simulink model "mpptPandO"  (R2024b)
settings: Solver=VariableStepAuto  StartTime=0.0  StopTime=1  RelTol=1e-3
undefined symbols (not defined in the file): sigbuilder_block
libraries: spsSeriesRLCBranchLib x4, spsCurrentMeasurementLib x1, spsDiodeLib x1, spsMosfetLib x1, spsPWMGeneratorDCDCLib x1, spsPVArrayLib x1, spsVoltageMeasurementLib x1, spspowerguiLib x1
settings Model: Creator=RASITH  LastModifiedBy=RASITH

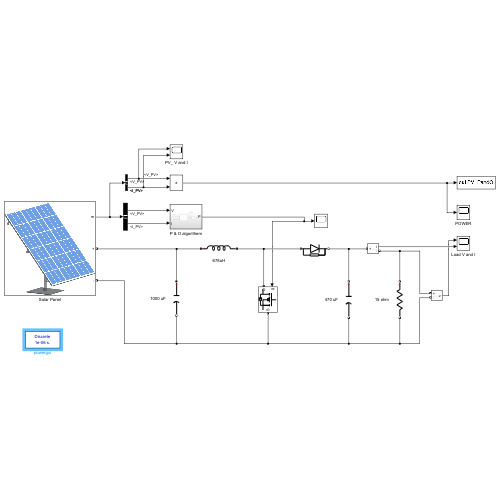
[thumbnail: Simulink's stored preview of the top-level diagram]
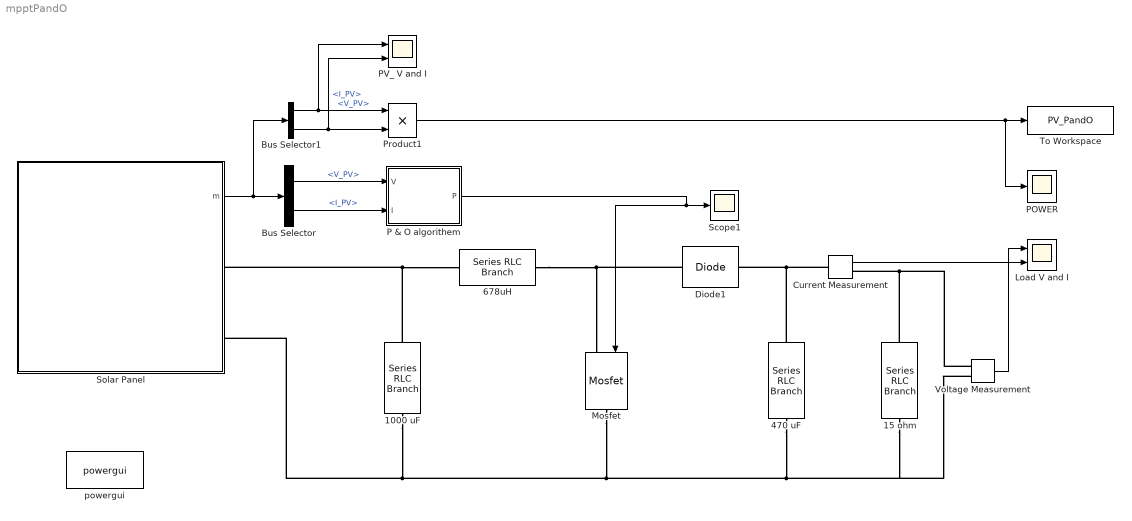
== system mpptPandO ==
  1000 uF : spsSeriesRLCBranchLib/Series RLC Branch  LConnTagsString=__new0  RConnTagsString=__new0  BranchType=C  Resistance=1  Inductance=1e-3  SetiL0=off  InitialCurrent=0  Capacitance=1e-3  Setx0=off  InitialVoltage=0  Measurements=None
  15 ohm : spsSeriesRLCBranchLib/Series RLC Branch  LConnTagsString=__new0  RConnTagsString=__new0  BranchType=R  Resistance=30  Inductance=1e-3  SetiL0=off  InitialCurrent=0  Capacitance=1e-6  Setx0=off  InitialVoltage=0  Measurements=None
  470 uF : spsSeriesRLCBranchLib/Series RLC Branch  LConnTagsString=__new0  RConnTagsString=__new0  BranchType=C  Resistance=1  Inductance=1e-3  SetiL0=off  InitialCurrent=0  Capacitance=470e-6  Setx0=off  InitialVoltage=0  Measurements=None
  678uH : spsSeriesRLCBranchLib/Series RLC Branch  LConnTagsString=__new0  RConnTagsString=__new0  BranchType=L  Resistance=1  Inductance=678e-6  SetiL0=off  InitialCurrent=0  Capacitance=1e-6  Setx0=off  InitialVoltage=0  Measurements=None
  Bus Selector : BusSelector  OutputSignals=V_PV,I_PV
  Bus Selector1 : BusSelector  OutputSignals=V_PV,I_PV
  Current Measurement : spsCurrentMeasurementLib/Current Measurement  PhasorSimulation=off  OutputType=Complex  PSBequivalent=0
  Diode1 : spsDiodeLib/Diode  Ron=0.001  Lon=0  Vf=0.8  IC=0  UseSnubber=0  Rs=500  Cs=250e-9  Measurements=off
  Load V and I : Scope  NumInputPorts=2
  Mosfet : spsMosfetLib/Mosfet  Ron=4.2e-3  Lon=0  Rd=0.01  Vfd=1  IC=0  Rs=1e5  Cs=1e-9  Measurements=off
  P & O algorithem : Subsystem
  POWER : Scope
  PV_ V and I : Scope  NumInputPorts=2
  Product1 : Product
  Scope1 : Scope
  Solar Panel : Subsystem
      mask Display: image('C:\Users\RASITH\MATLAB Drive\Final Year Project [MPPT Boost Converter(PV)]\Solar Panel.png');
  To Workspace : ToWorkspace  VariableName=PV_PandO  SaveFormat=Timeseries  SampleTime=-1
  Voltage Measurement : spsVoltageMeasurementLib/Voltage Measurement  PhasorSimulation=off  OutputType=Complex  PSBequivalent=0
  powergui : spspowerguiLib/powergui  Priority=1  SimulationMode=Discrete  SampleTime=1e-6  frequency=100000  Iterations=50  frequencyindice=0  Pbase=100e6  ErrMax=1e-4  UnitsV=kV  UnitsW=MW  buscounter=0  FunctionMessages=off  echomessages=off  EnableUseOfTLC=off  CurrentSourceSwitches=off  DisableSnubberDevices=off  DisableRonSwitches=off  DisableVfSwitches=off  DisplayEquations=off  AutomaticDiscreteSolvers=off  SolverType=Tustin/Backward Euler (TBE)  Interpol=off  ExternalGateDelay=off  methode=off  Ts=100  x0status=blocks  SPID=on  SwTol=0  HookPort=off  NonlinearTolerance=1e-4  nMaxIteration=100  ContinueOnMaxIteration=off  RestoreLinks=warning  ResistiveCurrentMeasurement=off  Frange=[0:2:500]  Ylog=off  Xlog=on  ShowGrid=off  save=off  variable=ZData  structure=0  ZoomFFT=off  StartTime=0.0  cycles=1  DisplayStyle=1  fundamental=60  FreqAxis=off  MaxFrequency=1000  frequencyindicesteady=1  RmsSteady=1  display=off
  wires:
  Solar Panel/1(m) -> Bus Selector1/1, Bus Selector/1
  Bus Selector/1 -> P & O algorithem/1(V)  "<V_PV>"
  Bus Selector/2 -> P & O algorithem/2(I)  "<I_PV>"
  Current Measurement/1 -> Load V and I/2
  Voltage Measurement/1 -> Load V and I/1
  Bus Selector1/1 -> PV_ V and I/1, Product1/1  "<V_PV>"
  Bus Selector1/2 -> Product1/2, PV_ V and I/2  "<I_PV>"
  Product1/1 -> To Workspace/1, POWER/1
  P & O algorithem/1(P) -> Scope1/1, Mosfet/1
  connections:
  1000 uF/RConn1 -- 15 ohm/RConn1 -- Voltage Measurement/LConn2 -- 470 uF/RConn1 -- Mosfet/RConn1 -- Solar Panel/RConn2
  678uH/RConn1 -- Diode1/LConn1 -- Mosfet/LConn1
  Current Measurement/LConn1 -- 470 uF/LConn1 -- Diode1/RConn1
  Voltage Measurement/LConn1 -- 15 ohm/LConn1 -- Current Measurement/RConn1
  1000 uF/LConn1 -- Solar Panel/RConn1 -- 678uH/LConn1

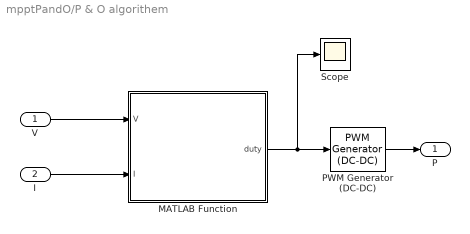
== system mpptPandO/P & O algorithem ==
  V : Inport
  I : Inport  Port=2
  MATLAB Function : MATLAB Function  TreatAsAtomicUnit=on
  PWM Generator (DC-DC) : spsPWMGeneratorDCDCLib/PWM Generator (DC-DC)  Fsw=10000  Ts=1e-6
  Scope : Scope
  P : Outport
  wires:
  I/1 -> MATLAB Function/2(I)
  V/1 -> MATLAB Function/1(V)
  PWM Generator (DC-DC)/1 -> P/1
  MATLAB Function/1(duty) -> PWM Generator (DC-DC)/1, Scope/1

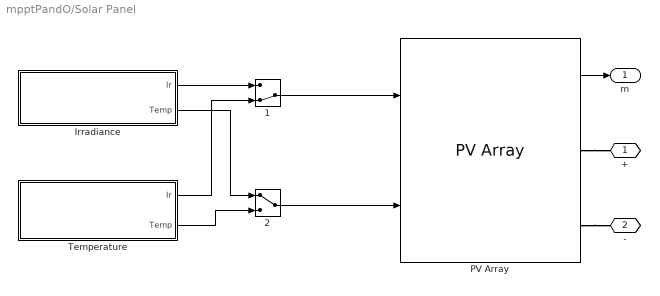
== system mpptPandO/Solar Panel ==
  "      1" : ManualSwitch  CurrentSetting=0
  "      2" : ManualSwitch
  "Irradiance " : Subsystem  Tag=STV Subsys  LoadFcn=sigbuilder_block('load');  StartFcn=sigbuilder_block('start');  StopFcn=sigbuilder_block('stop');  ClipboardFcn=sigbuilder_block('clipboard');  mask(Sigbuilder block){tuvar=[0:10]}
      mask help: Sigbuilder GUI
      mask init:
      | if ~strcmp(get_param(bdroot(gcbh),'SimulationStatus'),'stopped') tuvar = sigbuilder_block('maskInit'); end
      settings: CopyFcn=sigbuilder_block('copy');  DeleteFcn=sigbuilder_block('delete');  ModelCloseFcn=sigbuilder_block('modelClose');  PreSaveFcn=sigbuilder_block('preSave');  PauseFcn=sigbuilder_block('pause')  ContinueFcn=sigbuilder_block('continue')  NameChangeFcn=sigbuilder_block('namechange');  OpenFcn=sigbuilder_block('open',[5.4 30 1141.2 507.6 ]);  CloseFcn=sigbuilder_block('close');
      mask Display: plot(0, 0, 100, 100,[2, 2, 32, 32, 2], [68, 8, 8, 68, 68],[32, 2], [38, 38], [32, 19, 2],[53, 60, 44], [32, 17, 17, 2],[16, 16, 31, 31]);txt = getActiveGroup(gcbh);text(2, 100, txt,'verticalAlignment', 'top');
  PV Array : spsPVArrayLib/PV Array  Npar=1  Nser=1  PlotType=array @ 1000 W/m2 & specified temperatures  S_vec="[ 1000  500  100 ]"  Temp_C_vec="[ 25  ]"  ModuleName=User-defined  PlotWhenSelected=off  Pm=50.04  Ncell=36  Voc=23.4  Isc=2.92  Vm=18  Im=2.78  beta_Voc_pc=-0.36099  alpha_Isc_pc=0.102  beta_Voc=-0.084472  alpha_Isc=0.0029784  IL=2.9466  I0=1.0988e-10  nI=1.0538  Rsh=1848.6949  Rs=0.95616  RobustModel=off  RobustCellTemperature=313.3991  BAL=on  Tc=1e-6  Tfilter=5e-5
  Temperature : Subsystem  Tag=STV Subsys  LoadFcn=sigbuilder_block('load');  StartFcn=sigbuilder_block('start');  StopFcn=sigbuilder_block('stop');  ClipboardFcn=sigbuilder_block('clipboard');  mask(Sigbuilder block){tuvar=[0:10]}
      mask help: Sigbuilder GUI
      mask init:
      | if ~strcmp(get_param(bdroot(gcbh),'SimulationStatus'),'stopped') tuvar = sigbuilder_block('maskInit'); end
      settings: CopyFcn=sigbuilder_block('copy');  DeleteFcn=sigbuilder_block('delete');  ModelCloseFcn=sigbuilder_block('modelClose');  PreSaveFcn=sigbuilder_block('preSave');  PauseFcn=sigbuilder_block('pause')  ContinueFcn=sigbuilder_block('continue')  NameChangeFcn=sigbuilder_block('namechange');  OpenFcn=sigbuilder_block('open',[5.4 30 1141.2 507.6 ]);  CloseFcn=sigbuilder_block('close');
      mask Display: plot(0, 0, 100, 100,[2, 2, 32, 32, 2], [68, 8, 8, 68, 68],[32, 2], [38, 38], [32, 19, 2],[53, 60, 44], [32, 17, 17, 2],[16, 16, 31, 31]);txt = getActiveGroup(gcbh);text(2, 100, txt,'verticalAlignment', 'top');
  + : PMIOPort  Side=Right
  - : PMIOPort  Port=2  Side=Right
  m : Outport
  wires:
  "Irradiance "/1(Ir) -> "      1"/1
  "      2"/1 -> PV Array/2
  "      1"/1 -> PV Array/1
  Temperature/2(Temp) -> "      2"/2
  Temperature/1(Ir) -> "      1"/2
  "Irradiance "/2(Temp) -> "      2"/1
  PV Array/1 -> m/1
  connections:
  PV Array/RConn1 -- +/RConn1
  PV Array/RConn2 -- -/RConn1

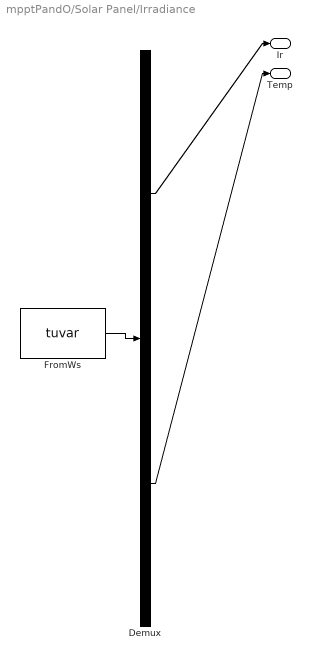
== system mpptPandO/Solar Panel/Irradiance  ==
  Demux : Demux  Tag=STV Demux  Outputs=2
      settings: DisplayOption=none
  FromWs : FromWorkspace  Tag=STV FromWs  VariableName=tuvar
      SigBuilderData=|
      | common.afterFinalStr = 'Extrapolate'
      | common.sampleTime = '0'
      | dataSet(1).timeRange = [0 2]
      | dataSet(1).name = 'Constant Irradiance'
      | dataSet(2).timeRange = [0 2]
      | dataSet(2).name = 'Step Irradiance'
      | dataSet(3).timeRange = [0 1]
      | dataSet(3).name = 'Ramp-up/down Irradiance'
      | sbobj.Groups(1).Name = 'Constant Irradiance'
      | sbobj.Groups(1).Signals(1).Name = 'Ir'
      | sbobj.Groups(1).Signals(1).XData = [0 2]
      | sbobj.Groups(1).Signals(1).YData = [1000 1000]
      | sbobj.Groups(1).Signals(2).Name = 'Temp'
      | sbobj.Groups(1).Signals(2).XData = [0 1 1 2]
      | sbobj.Groups(1).Signals(2).YData = [0 0 1 1]
      | sbobj.Groups(1).TimeRange = [0 2]
      | sbobj.Groups(2).Name = 'Step Irradiance'
      | sbobj.Groups(2).Signals(1).Name = 'Ir'
      | sbobj.Groups(2).Signals(1).XData = [0 0.252 0.252 2]
      | sbobj.Groups(2).Signals(1).YData = [600 600 1000 1000]
      | sbobj.Groups(2).Signals(2).Name = 'Temp'
      | sbobj.Groups(2).Signals(2).XData = [0 1 1 2]
      | sbobj.Groups(2).Signals(2).YData = [0 0 1 1]
      | sbobj.Groups(2).TimeRange = [0 2]
      | sbobj.Groups(3).Name = 'Ramp-up/down Irradiance'
      | sbobj.Groups(3).Signals(1).Name = 'Ir'
      | sbobj.Groups(3).Signals(1).XData = [0 0.2 0.2 0.4 0.4 0.6 0.6 0.8 0.8 1]
      | sbobj.Groups(3).Signals(1).YData = [200 200 400 400 600 600 800 800 1000 1000]
      | sbobj.Groups(3).Signals(2).Name = 'Temp'
      | sbobj.Groups(3).Signals(2).XData = [0 1]
      | sbobj.Groups(3).Signals(2).YData = [25 25]
      | sbobj.Groups(3).TimeRange = [0 1]
  Ir : Outport  Tag=STV Outport
  Temp : Outport  Tag=STV Outport  Port=2
  wires:
  Demux/1 -> Ir/1
  FromWs/1 -> Demux/1
  Demux/2 -> Temp/1

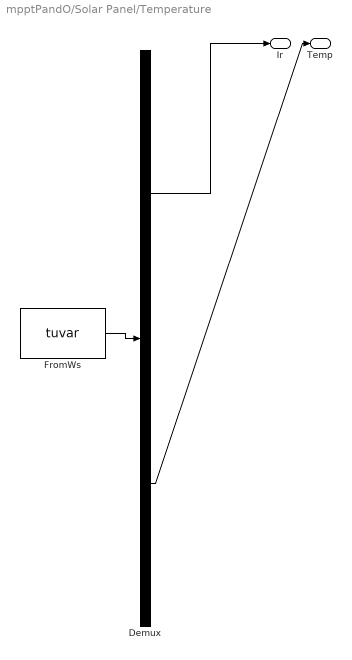
== system mpptPandO/Solar Panel/Temperature ==
  Demux : Demux  Tag=STV Demux  Outputs=2
      settings: DisplayOption=none
  FromWs : FromWorkspace  Tag=STV FromWs  VariableName=tuvar
      SigBuilderData=|
      | common.afterFinalStr = 'Extrapolate'
      | common.sampleTime = '0'
      | dataSet(1).timeRange = [0 2]
      | dataSet(1).name = 'Constant Irradiance'
      | dataSet(2).timeRange = [0 2]
      | dataSet(2).name = 'Ramp-up/down Irradiance'
      | dataSet(3).timeRange = [0 2]
      | dataSet(3).name = 'Step Irradiance'
      | sbobj.Groups(1).Name = 'Constant Irradiance'
      | sbobj.Groups(1).Signals(1).Name = 'Ir'
      | sbobj.Groups(1).Signals(1).XData = [0 2]
      | sbobj.Groups(1).Signals(1).YData = [1000 1000]
      | sbobj.Groups(1).Signals(2).Name = 'Temp'
      | sbobj.Groups(1).Signals(2).XData = [0 0.398 0.398 0.8 0.8 1.2 1.2 1.6 1.6 2]
      | sbobj.Groups(1).Signals(2).YData = [15 15 25 25 39 39 60 60 75 75]
      | sbobj.Groups(1).TimeRange = [0 2]
      | sbobj.Groups(2).Name = 'Ramp-up/down Irradiance'
      | sbobj.Groups(2).Signals(1).Name = 'Ir'
      | sbobj.Groups(2).Signals(1).XData = [0 0.3 0.3 0.4 0.4 0.5 0.5 1 2]
      | sbobj.Groups(2).Signals(1).YData = [1000 1000 800 795 600 600 400 395 395]
      | sbobj.Groups(2).Signals(2).Name = 'Temp'
      | sbobj.Groups(2).Signals(2).XData = [0 0.8 0.8 2]
      | sbobj.Groups(2).Signals(2).YData = [15 15 35 35]
      | sbobj.Groups(2).TimeRange = [0 2]
      | sbobj.Groups(3).Name = 'Step Irradiance'
      | sbobj.Groups(3).Signals(1).Name = 'Ir'
      | sbobj.Groups(3).Signals(1).XData = [0 0.252 0.252 2]
      | sbobj.Groups(3).Signals(1).YData = [600 600 1000 1000]
      | sbobj.Groups(3).Signals(2).Name = 'Temp'
      | sbobj.Groups(3).Signals(2).XData = [0 0.6 0.6 2]
      | sbobj.Groups(3).Signals(2).YData = [15 15 36.5 19.5]
      | sbobj.Groups(3).TimeRange = [0 2]
  Ir : Outport  Tag=STV Outport
  Temp : Outport  Tag=STV Outport  Port=2
  wires:
  FromWs/1 -> Demux/1
  Demux/1 -> Ir/1
  Demux/2 -> Temp/1

== matlab function mpptPandO/P & O algorithem/MATLAB Function ==
  data: V input; duty output; I input
function duty = PandO_Algorithm(V, I)
    % Stabilized P&O MPPT Algorithm
    % Includes Execution Delay and Deadband
    
    persistent V_old P_old D_old Loop_Counter;

    % Initialization
    if isempty(D_old)
        V_old = 0;
        P_old = 0;
        D_old = 0.29;   % Start near the expected 29% to reduce startup swing
        Loop_Counter = 0;
    end

    % --- TUNING PARAMETERS ---
    % 1. Step Size: Smaller steps reduce oscillation magnitude
    deltaD = 0.002;   
    
    % 2. Update Delay: How many simulation steps to wait before changing Duty.
    % Increase this if oscillation continues. (Try 500, 1000, or 2000)
    Update_Delay = 500; 
    
    % 3. Power Deadband: Ignore tiny power changes (noise)
    Power_Deadband = 0.2; % Watts

    % --- Code Execution ---
    P = V * I;
    Loop_Counter = Loop_Counter + 1;

    % CHECK: Only run P&O logic if the delay time has passed
    if Loop_Counter >= Update_Delay
        
        % Reset Counter
        Loop_Counter = 0;
        
        dP = P - P_old;
        dV = V - V_old;

        % Only change Duty if power change is real (larger than deadband)
        if abs(dP) > Power_Deadband
            if dP > 0
                % Power INCREASED
                if dV > 0
                    D_old = D_old - deltaD; % Left of MPP -> Decrease D (Increase V)
                else
                    D_old = D_old + deltaD; % Right of MPP -> Increase D (Decrease V)
                end
            else
                % Power DECREASED
                if dV > 0
                    D_old = D_old + deltaD; % Go back
                else
                    D_old = D_old - deltaD; % Go back
                end
            end
        end
        
        % Saturation Limits
        if D_old > 0.85
            D_old = 0.85;
        elseif D_old < 0.05
            D_old = 0.05;
        end
        
        % Update History only when we actually calculate
        V_old = V;
        P_old = P;
    end

    % Output the held Duty Cycle
    duty = D_old;
end
